simulink model "inertia"  (R2022b)
settings: Solver=ode5  StartTime=0.0  StopTime=t_s  FixedStep=h  RelTol=1e-3
undefined symbols (not defined in the file): J, K
libraries: simulink x2
settings Model: Creator=Claudia  LastModifiedBy=Claudia Yasar
settings SolverCC: AlgebraicLoopSolver=TrustRegion
settings DataIOCC: ReturnWorkspaceOutputs=off
settings DebuggingCC: UnconnectedInputMsg=warning  UnconnectedOutputMsg=warning  UnconnectedLineMsg=warning  SFMachineParentedDataDiag=warning  ArithmeticOperatorsInVariantConditions=warning
settings ModelReferenceCC: EnableRefExpFcnMdlSchedulingChecks=on
settings SFSimCC: CustomCodeUndefinedFunction=UseInterfaceOnly

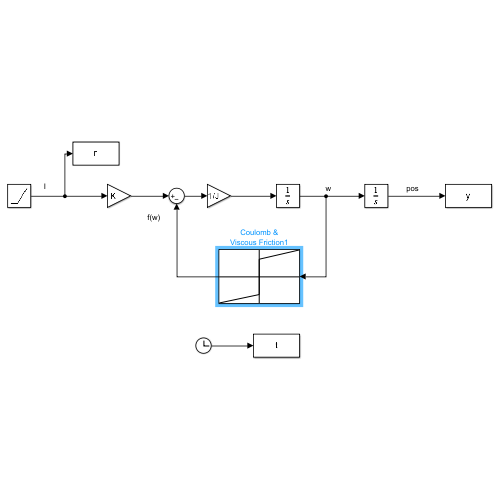
[thumbnail: Simulink's stored preview of the top-level diagram]
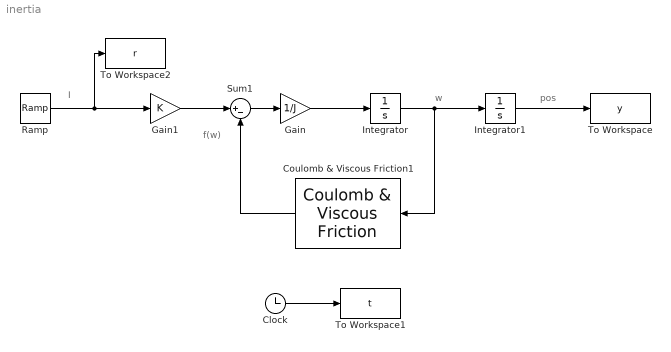
== system inertia ==
  note: I
  note: pos
  note: w
  note: f(w)
  Clock : Clock
  Coulomb & Viscous Friction1 : simulink/Discontinuities/Coulomb & Viscous Friction  offset=2  gain=1
  Gain : Gain  Gain=1/J
  Gain1 : Gain  Gain=K
  Integrator : Integrator
  Integrator1 : Integrator
  Ramp : simulink/Sources/Ramp  slope=1  start=0  InitialOutput=0
  Sum1 : Sum  Inputs=|+-
  To Workspace : ToWorkspace  VariableName=y  SampleTime=-1
      settings: OpenFcn=figure;plot(t,y);
  To Workspace1 : ToWorkspace  VariableName=t  SampleTime=-1
  To Workspace2 : ToWorkspace  VariableName=r  SampleTime=-1
      settings: OpenFcn=figure;plot(t,y);
  wires:
  Clock/1 -> To Workspace1/1
  Ramp/1 -> Gain1/1, To Workspace2/1
  Gain/1 -> Integrator/1
  Integrator1/1 -> To Workspace/1
  Integrator/1 -> Coulomb & Viscous Friction1/1, Integrator1/1
  Sum1/1 -> Gain/1
  Gain1/1 -> Sum1/1
  Coulomb & Viscous Friction1/1 -> Sum1/2
